simulink model "tower_mpc"  (Simulink 8.6)
settings: Solver=VariableStepDiscrete  StartTime=0.0  StopTime=10.0  RelTol=1e-3
undefined symbols (not defined in the file): tower, tower_x0, tower_xref, Ts
libraries: mpclib x1
settings Model: Creator=matias  LastModifiedBy=pdoren
settings DebuggingCC: FcnCallInpInsideContextMsg=EnableAllAsWarning

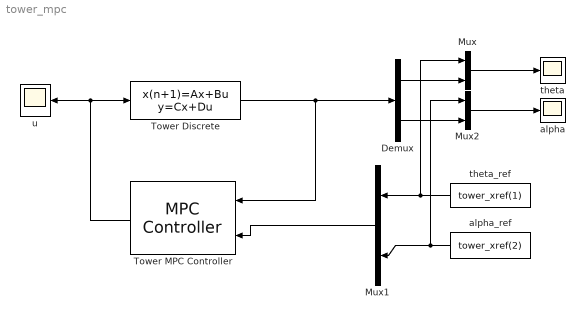
== system tower_mpc ==
  Demux : Demux  Outputs=2
  Mux : Mux  Inputs=2
  Mux1 : Mux  Inputs=2
  Mux2 : Mux  Inputs=2
  Tower Discrete : DiscreteStateSpace  A=tower.A  B=tower.B  C=tower.C  D=tower.D  X0=tower_x0  SampleTime=Ts
  Tower MPC Controller : mpclib/MPC Controller  mpcobj=tower_MPC  x0=[]  is_multiple=0  enable_value=0  return_u0=off  ref_from_ws=off  ref_signal_name=[]  ref_preview=on  md_from_ws=off  md_signal_name=[]  md_preview=on  from_project=off  project_file=MPCtask.mat  md_inport=off  mv_inport=off  cost_outport=off  return_sequence=off  return_qpstatus=off  return_state=off  state_inport=off  lims_inport=off  ywt_inport=off  is_designfromscratch=0  uwt_inport=off  duwt_inport=off  rhoeps_inport=off  uref_inport=off  n_ts=0.05  n_mv=1  n_md=0  n_ud=0  n_mo=2  n_uo=0  BlockDataType=double  SampleTimeInherited=off  switch_inport=off
  alpha : Scope
  alpha_ref : Constant  Value=tower_xref(2)
  theta : Scope
  theta_ref : Constant  Value=tower_xref(1)
  u : Scope
  wires:
  Tower Discrete/1 -> Demux/1, Tower MPC Controller/1
  Tower MPC Controller/1 -> Tower Discrete/1, u/1
  Mux/1 -> theta/1
  theta_ref/1 -> Mux/1, Mux1/1
  Mux1/1 -> Tower MPC Controller/2
  Mux2/1 -> alpha/1
  Demux/1 -> Mux/2
  alpha_ref/1 -> Mux1/2, Mux2/1
  Demux/2 -> Mux2/2
